simulink model "PI_VSRPhysicalModel"  (R2021a)
settings: Solver=ode23  StartTime=0.0  StopTime=.2  FixedStep=1e-6  MaxStep=1e-6  RelTol=1e-3
InitFcn:
  | Ts = 1e-6;
  | f_PWM = 20000;
  | tf = f_PWM * Ts;
  | L = 2e-3;
  | omega = 2*pi*50;
  | a = exp(1i*2*pi/3);
  | R = 0.5;
  | C  = 1500e-6;
  | tau_c = 7.95e-05;
  | kp = L/tau_c;
  | ki = R/tau_c;
undefined symbols (not defined in the file): DiscIntNeverNeededParam
libraries: pid_lib x5, spsabctodq0Lib x4, spsControlledVoltageSourceLib x3, spsSeriesRLCBranchLib x2, spsdq0toAlphaBetaZeroLib x2, spsGroundLib x1, spsThreePhaseVIMeasurementLib x1, simulink x1, mcbcontrolslib x1, spsThreePhaseSeriesRLCBranchLib x1, spsUniversalBridgeLib x1, spsVoltageMeasurementLib x1
settings Model: Creator=Kibrom  LastModifiedBy=Kibrom

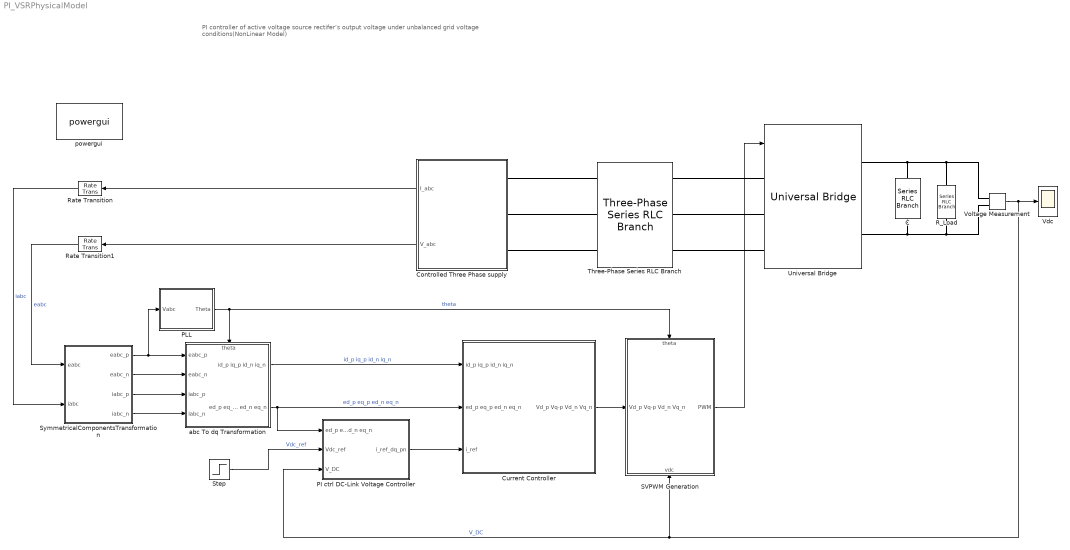
== system PI_VSRPhysicalModel ==
  note: PI controller of active voltage source rectifer’s output voltage under unbalanced grid voltage conditions(NonLinear Model)
  C : spsSeriesRLCBranchLib/Series RLC Branch  LConnTagsString=__new0  RConnTagsString=__new0  BranchType=C  Resistance=1  Inductance=1e-3  SetiL0=off  InitialCurrent=0  Capacitance=1500e-6  Setx0=on  InitialVoltage=650  Measurements=None
  Controlled Three Phase supply : Subsystem
      settings: PortSchema="{\"entries\":[{\"content\":{\"sides\":[{\"content\":{\"connectorIds\":[\"Out1\",\"Out2\"]},\"type\":\"ConnectorPlacement.EquallySpacedRectSide\",\"uuid\":\"e5d84f7a-0d8d-41f6-8cc2-6d81f08370fc\"},{\"content\":{\"connectorIds\":[\"RConn1\",\"RConn2\",\"RConn3\"],\"side\":\"RIGHT\"},\"type\":\"ConnectorPlacement.EquallySpacedRectSide\",\"uuid\":\"372d453a-1c29-4369-a80d-bd12301de137\"},{\"content\":{\"connectorIds\":[],\"side\":\"TOP\"},\"type\":\"ConnectorPlacement.EquallySpacedRectSide\",\"uuid\":\"f7f34885-8130-4d5d-8b71-b12e9f31364c\"}]},\"type\":\"ConnectorPlacement.EquallySpacedConnector\",\"uuid\":\"3797b9c2-a6ae-4ab8-888b-5dd066a2b1e3\"}],\"packageUris\":[\"http://schema.mathworks.com/mf0/Connector/R2020b\"],\"version\":\"1.0\"}"
  Current Controller : Subsystem
  PI ctrl DC-Link Voltage Controller : Subsystem
  PLL : Subsystem
  R_Load : spsSeriesRLCBranchLib/Series RLC Branch  LConnTagsString=__new0  RConnTagsString=__new0  BranchType=R  Resistance=60  Inductance=1e-3  SetiL0=off  InitialCurrent=0  Capacitance=1e-6  Setx0=off  InitialVoltage=0  Measurements=None
  Rate Transition : RateTransition  OutPortSampleTime=5e-5
  Rate Transition1 : RateTransition  OutPortSampleTime=5e-5
  SVPWM Generation : Subsystem
      settings: PortSchema="{\"entries\":[{\"content\":{\"sides\":[{\"content\":{\"connectorIds\":[\"In1\"]},\"type\":\"ConnectorPlacement.EquallySpacedRectSide\",\"uuid\":\"b01bcb52-9446-408f-a811-167d66cc3532\"},{\"content\":{\"connectorIds\":[\"Out1\"],\"side\":\"RIGHT\"},\"type\":\"ConnectorPlacement.EquallySpacedRectSide\",\"uuid\":\"648c50fb-9991-4e3a-92fd-e8050aaa738b\"},{\"content\":{\"connectorIds\":[\"In2\"],\"side\":\"TOP\"},\"type\":\"ConnectorPlacement.EquallySpacedRectSide\",\"uuid\":\"7ec30d75-e250-4e03-a8de-fbe51cb0d640\"},{\"content\":{\"connectorIds\":[\"In3\"],\"side\":\"BOTTOM\"},\"type\":\"ConnectorPlacement.EquallySpacedRectSide\",\"uuid\":\"2bac38e0-cfd2-4a7e-a696-b4a008d5ca86\"}]},\"type\":\"ConnectorPlacement.EquallySpacedConnector\",\"uuid\":\"00db0e70-35b6-41ae-bea5-41b2b525dd01\"}],\"packageUris\":[\"http://schema.mathworks.com/mf0/Connector/R2020b\"],\"version\":\"1.0\"}"
  Step : Step  Time=0.1  Before=650  After=700  SampleTime=5e-04
  SymmetricalComponentsTransformation : Subsystem
  Three-Phase Series RLC Branch : spsThreePhaseSeriesRLCBranchLib/Three-Phase Series RLC Branch  LConnTagsString=A|B|C  RConnTagsString=A|B|C  BranchType=RL  Resistance=R  Inductance=2*L  Capacitance=1e-6  Measurements=None
  Universal Bridge : spsUniversalBridgeLib/Universal Bridge  Arms=3  SnubberResistance=1e5  SnubberCapacitance=inf  Device=IGBT / Diodes  Ron=1e-3  Lon=0  ForwardVoltages="[  0  0  ]"  ForwardVoltage=0  GTOparameters=[ 10e-6 , 20e-6 ]  IGBTparameters=[ 1e-6 , 2e-6 ]  Measurements=None  Measurements_2=None  converterType=Rectifier
  Vdc : Scope
  Voltage Measurement : spsVoltageMeasurementLib/Voltage Measurement  PhasorSimulation=off  OutputType=Complex  PSBequivalent=0
  abc To dq Transformation : Subsystem
      settings: PortSchema="{\"entries\":[{\"content\":{\"sides\":[{\"content\":{\"connectorIds\":[\"In1\",\"In2\",\"In3\",\"In4\"]},\"type\":\"ConnectorPlacement.EquallySpacedRectSide\",\"uuid\":\"dcaee8e7-dac1-4a7e-bdf9-5644c9a478e5\"},{\"content\":{\"connectorIds\":[\"Out1\",\"Out2\"],\"side\":\"RIGHT\"},\"type\":\"ConnectorPlacement.EquallySpacedRectSide\",\"uuid\":\"35135458-27d9-4a99-822f-710c0f77fa66\"},{\"content\":{\"connectorIds\":[\"In5\"],\"side\":\"TOP\"},\"type\":\"ConnectorPlacement.EquallySpacedRectSide\",\"uuid\":\"74ffbf0c-7c15-41c6-8afa-503588a6e7a3\"}]},\"type\":\"ConnectorPlacement.EquallySpacedConnector\",\"uuid\":\"51b18d8e-0b4d-44db-b422-35434fbd35e0\"}],\"packageUris\":[\"http://schema.mathworks.com/mf0/Connector/R2020b\"],\"version\":\"1.0\"}"
  powergui : spspowerguiLib/powergui  Priority=1  SimulationMode=Discrete  SampleTime=Ts  frequency=60  Iterations=50  frequencyindice=0  Pbase=100e6  ErrMax=1e-4  UnitsV=kV  UnitsW=MW  buscounter=0  FunctionMessages=off  echomessages=off  EnableUseOfTLC=off  CurrentSourceSwitches=off  DisableSnubberDevices=off  DisableRonSwitches=off  DisableVfSwitches=off  DisplayEquations=off  AutomaticDiscreteSolvers=off  SolverType=Tustin/Backward Euler (TBE)  Interpol=off  ExternalGateDelay=off  methode=off  Ts=100  x0status=blocks  SPID=on  SwTol=0  HookPort=off  NonlinearTolerance=1e-4  nMaxIteration=100  ContinueOnMaxIteration=off  RestoreLinks=warning  ResistiveCurrentMeasurement=off  Frange=[0:2:500]  Ylog=off  Xlog=on  ShowGrid=off  save=off  variable=ZData  structure=0  ZoomFFT=off  StartTime=0.0  cycles=1  DisplayStyle=1  fundamental=60  FreqAxis=off  MaxFrequency=1000  frequencyindicesteady=1  RmsSteady=1  display=off
  wires:
  SVPWM Generation/1(PWM) -> Universal Bridge/1
  PLL/1(Theta) -> SVPWM Generation/2(theta), abc To dq Transformation/5(theta)  "theta"
  Voltage Measurement/1 -> PI ctrl DC-Link Voltage Controller/3(V_DC), SVPWM Generation/3(vdc), Vdc/1  "V_DC"
  Rate Transition1/1 -> SymmetricalComponentsTransformation/1(eabc)  "eabc"
  Current Controller/1(Vd_p Vq-p Vd_n Vq_n) -> SVPWM Generation/1(Vd_p Vq-p Vd_n Vq_n)
  abc To dq Transformation/1(id_p iq_p id_n iq_n) -> Current Controller/1(id_p iq_p id_n iq_n)  "id_p iq_p id_n iq_n"
  abc To dq Transformation/2(ed_p eq_p ed_n eq_n) -> PI ctrl DC-Link Voltage Controller/1(ed_p eq_p ed_n eq_n), Current Controller/2(ed_p eq_p ed_n eq_n)  "ed_p eq_p ed_n eq_n"
  Rate Transition/1 -> SymmetricalComponentsTransformation/2(iabc)  "iabc"
  Controlled Three Phase supply/1(I_abc) -> Rate Transition/1
  Controlled Three Phase supply/2(V_abc) -> Rate Transition1/1
  SymmetricalComponentsTransformation/1(eabc_p) -> PLL/1(Vabc), abc To dq Transformation/1(eabc_p)
  SymmetricalComponentsTransformation/4(iabc_n) -> abc To dq Transformation/4(iabc_n)
  SymmetricalComponentsTransformation/3(iabc_p) -> abc To dq Transformation/3(iabc_p)
  SymmetricalComponentsTransformation/2(eabc_n) -> abc To dq Transformation/2(eabc_n)
  Step/1 -> PI ctrl DC-Link Voltage Controller/2(Vdc_ref)  "Vdc_ref"
  PI ctrl DC-Link Voltage Controller/1(i_ref_dq_pn) -> Current Controller/3(i_ref)
  connections:
  Voltage Measurement/LConn2 -- Universal Bridge/RConn2 -- C/RConn1 -- R_Load/RConn1
  Universal Bridge/LConn1 -- Three-Phase Series RLC Branch/RConn1
  Universal Bridge/LConn2 -- Three-Phase Series RLC Branch/RConn2
  Universal Bridge/LConn3 -- Three-Phase Series RLC Branch/RConn3
  Universal Bridge/RConn1 -- R_Load/LConn1 -- Voltage Measurement/LConn1 -- C/LConn1
  Controlled Three Phase supply/RConn1 -- Three-Phase Series RLC Branch/LConn1
  Controlled Three Phase supply/RConn2 -- Three-Phase Series RLC Branch/LConn2
  Controlled Three Phase supply/RConn3 -- Three-Phase Series RLC Branch/LConn3

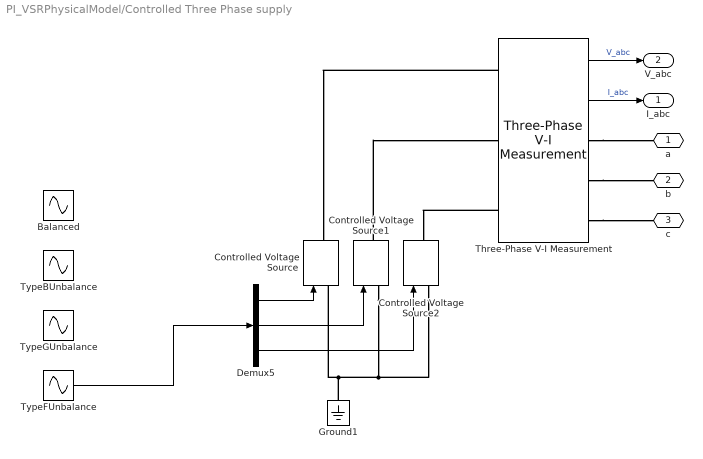
== system PI_VSRPhysicalModel/Controlled Three Phase supply ==
  Balanced : Sin  Amplitude=sqrt(2)*[230 230 230]  Frequency=2*pi*50  Phase=[0 240 120]*(pi/180)  SampleTime=0
  Controlled Voltage Source : spsControlledVoltageSourceLib/Controlled Voltage Source  Initialize=on  Source_Type=AC  Amplitude=0  Phase=0  Frequency=0  Measurements=None
  Controlled Voltage Source1 : spsControlledVoltageSourceLib/Controlled Voltage Source  Initialize=on  Source_Type=AC  Amplitude=0  Phase=0  Frequency=0  Measurements=None
  Controlled Voltage Source2 : spsControlledVoltageSourceLib/Controlled Voltage Source  Initialize=on  Source_Type=AC  Amplitude=0  Phase=0  Frequency=0  Measurements=None
  Demux5 : Demux  Outputs=3
  Ground1 : spsGroundLib/Ground  LConnTagsString=a
  Three-Phase V-I Measurement : spsThreePhaseVIMeasurementLib/Three-Phase V-I Measurement  VoltageMeasurement=phase-to-ground  SetLabelV=off  LabelV=Vabc  Vpu=off  VpuLL=off  CurrentMeasurement=yes  SetLabelI=off  LabelI=Iabc  Ipu=off  Pbase=100e6  Vbase=500e3  OutputType=Complex  PhasorSimulation=off  PSBequivalent=0
  TypeBUnbalance : Sin  Amplitude=sqrt(2)*[185 230 230]  Frequency=2*pi*50  Phase=[0 240 120]*(pi/180)  SampleTime=0
  TypeFUnbalance : Sin  Amplitude=sqrt(2)*[184 207.4 207.4]  Frequency=2*pi*50  Phase=[0 243.7 116.3]*(pi/180)  SampleTime=0
  TypeGUnbalance : Sin  Amplitude=sqrt(2)*[214.6 192.1 192.1]  Frequency=2*pi*50  Phase=[0 236 124]*(pi/180)  SampleTime=0
  a : PMIOPort  Side=Right
  b : PMIOPort  Port=2  Side=Right
  c : PMIOPort  Port=3  Side=Right
  I_abc : Outport
  V_abc : Outport  Port=2
  wires:
  TypeFUnbalance/1 -> Demux5/1
  Three-Phase V-I Measurement/2 -> I_abc/1  "I_abc"
  Demux5/2 -> Controlled Voltage Source1/1
  Demux5/3 -> Controlled Voltage Source2/1
  Demux5/1 -> Controlled Voltage Source/1
  Three-Phase V-I Measurement/1 -> V_abc/1  "V_abc"
  connections:
  Controlled Voltage Source1/RConn1 -- Three-Phase V-I Measurement/LConn2
  Controlled Voltage Source/LConn1 -- Ground1/LConn1 -- Controlled Voltage Source1/LConn1 -- Controlled Voltage Source2/LConn1
  Three-Phase V-I Measurement/LConn3 -- Controlled Voltage Source2/RConn1
  Three-Phase V-I Measurement/LConn1 -- Controlled Voltage Source/RConn1
  Three-Phase V-I Measurement/RConn3 -- c/RConn1
  Three-Phase V-I Measurement/RConn1 -- a/RConn1
  Three-Phase V-I Measurement/RConn2 -- b/RConn1

== system PI_VSRPhysicalModel/Current Controller ==
  id_p iq_p id_n iq_n : Inport
  ed_p eq_p ed_n eq_n : Inport  Port=2
  i_ref : Inport  Port=3
  Demux : Demux
  Demux1 : Demux  Outputs=2
  Demux2 : Demux  Outputs=2
  Mux : Mux
  NegatveSeq Current Controller : Subsystem
      settings: PortSchema="{\"entries\":[{\"content\":{\"sides\":[{\"content\":{\"connectorIds\":[\"In1\",\"In2\",\"In3\"]},\"type\":\"ConnectorPlacement.EquallySpacedRectSide\",\"uuid\":\"2bdf4aa8-c3f9-436b-9835-043d932fea71\"},{\"content\":{\"connectorIds\":[\"Out1\",\"Out2\"],\"side\":\"RIGHT\"},\"type\":\"ConnectorPlacement.EquallySpacedRectSide\",\"uuid\":\"c965a7a2-5936-47cc-8492-850bd324378e\"},{\"content\":{\"connectorIds\":[],\"side\":\"TOP\"},\"type\":\"ConnectorPlacement.EquallySpacedRectSide\",\"uuid\":\"45debca4-d3b7-48eb-be8d-4eccd646cb24\"},{\"content\":{\"connectorIds\":[\"In4\"],\"side\":\"BOTTOM\"},\"type\":\"ConnectorPlacement.EquallySpacedRectSide\",\"uuid\":\"6975aea9-83b3-4c6b-a4f1-94e60a0e1fe9\"}]},\"type\":\"ConnectorPlacement.EquallySpacedConnector\",\"uuid\":\"b897b5d1-f6c9-41b8-aee6-e6cc6417929b\"}],\"packageUris\":[\"http://schema.mathworks.com/mf0/Connector/R2020b\"],\"version\":\"1.0\"}"
  PostiveSeq Current Controller : Subsystem
      settings: PortSchema="{\"entries\":[{\"content\":{\"sides\":[{\"content\":{\"connectorIds\":[\"In1\",\"In2\",\"In3\"]},\"type\":\"ConnectorPlacement.EquallySpacedRectSide\",\"uuid\":\"2bdf4aa8-c3f9-436b-9835-043d932fea71\"},{\"content\":{\"connectorIds\":[\"Out1\",\"Out2\"],\"side\":\"RIGHT\"},\"type\":\"ConnectorPlacement.EquallySpacedRectSide\",\"uuid\":\"c965a7a2-5936-47cc-8492-850bd324378e\"},{\"content\":{\"connectorIds\":[\"In4\"],\"side\":\"TOP\"},\"type\":\"ConnectorPlacement.EquallySpacedRectSide\",\"uuid\":\"45debca4-d3b7-48eb-be8d-4eccd646cb24\"}]},\"type\":\"ConnectorPlacement.EquallySpacedConnector\",\"uuid\":\"b897b5d1-f6c9-41b8-aee6-e6cc6417929b\"}],\"packageUris\":[\"http://schema.mathworks.com/mf0/Connector/R2020b\"],\"version\":\"1.0\"}"
  Vd_p Vq-p Vd_n Vq_n : Outport
  wires:
  Demux1/1 -> PostiveSeq Current Controller/1(id_p iq_p)  "id_p iq_p"
  Demux/3 -> NegatveSeq Current Controller/1(id_ref)
  Demux2/2 -> NegatveSeq Current Controller/4(ed_n eq_n)  "ed_n eq_n"
  PostiveSeq Current Controller/1(Vd_p) -> Mux/1
  Demux2/1 -> PostiveSeq Current Controller/4(ed_p eq_p)  "ed_p eq_p"
  Demux/4 -> NegatveSeq Current Controller/2(iq_ref)
  NegatveSeq Current Controller/1(Vd_n) -> Mux/3
  NegatveSeq Current Controller/2(Vq_n) -> Mux/4
  Demux/1 -> PostiveSeq Current Controller/2(id_ref)
  Demux/2 -> PostiveSeq Current Controller/3(iq_ref)
  PostiveSeq Current Controller/2(Vq_p) -> Mux/2
  Demux1/2 -> NegatveSeq Current Controller/3(id_n iq_n)  "id_n iq_n"
  Mux/1 -> Vd_p Vq-p Vd_n Vq_n/1  "Vd_p Vq-p Vd_n Vq_n"
  i_ref/1 -> Demux/1
  id_p iq_p id_n iq_n/1 -> Demux1/1
  ed_p eq_p ed_n eq_n/1 -> Demux2/1

== system PI_VSRPhysicalModel/PI ctrl DC-Link Voltage Controller ==
  ed_p eq_p ed_n eq_n : Inport
  Vdc_ref : Inport  Port=2
  V_DC : Inport  Port=3
  MATLAB Function : MATLAB Function  TreatAsAtomicUnit=on
  PID Controller : pid_lib/PID Controller  Controller=PID  Form=Parallel  TimeDomain=Continuous-time  UseExternalTs=off  SampleTime=-1  IntegratorMethod=Forward Euler  FilterMethod=Forward Euler  ControllerParametersSource=internal  P=1  I=1  D=0  UseFilter=on  N=100  TunerSelectOption=Transfer Function Based (PID Tuner App)  InitialConditionSource=internal  InitialConditionForIntegrator=0  InitialConditionForFilter=0  DifferentiatorICPrevScaledInput=0  ExternalReset=none  TrackingMode=off  Kt=1  LimitOutput=off  SatLimitsSource=internal  UpperSaturationLimit=inf  LowerSaturationLimit=-inf  LinearizeAsGain=on  AntiWindupMode=none  Kb=1  POutMin=[]  POutMax=[]  IOutMin=[]  IOutMax=[]  DOutMin=[]  DOutMax=[]  NOutMin=[]  NOutMax=[]  SumOutMin=[]  SumOutMax=[]  SaturationOutMin=[]  SaturationOutMax=[]  PParamMin=[]  PParamMax=[]  IParamMin=[]  IParamMax=[]  DParamMin=[]  DParamMax=[]  NParamMin=[]  NParamMax=[]  KbParamMin=[]  KbParamMax=[]  KtParamMin=[]  KtParamMax=[]  KbOutMin=[]  KbOutMax=[]  KtOutMin=[]  KtOutMax=[]  IntegratorOutMin=[]  IntegratorOutMax=[]  FilterOutMin=[]  FilterOutMax=[]  SumI1OutMin=[]  SumI1OutMax=[]  SumI2OutMin=[]  SumI2OutMax=[]  SumI3OutMin=[]  SumI3OutMax=[]  SumI4OutMin=[]  SumI4OutMax=[]  SumDOutMin=[]  SumDOutMax=[]  DifferentiatorOutMin=[]  DifferentiatorOutMax=[]  FilterDiffOutCoefMin=[]  FilterDiffOutCoefMax=[]  ReciprocalOutMin=[]  ReciprocalOutMax=[]  SumDenOutMin=[]  SumDenOutMax=[]  SumNumOutMin=[]  SumNumOutMax=[]  DivideOutMin=[]  DivideOutMax=[]  UdiffTsProdOutMin=[]  UdiffTsProdOutMax=[]  NTsProdOutMin=[]  NTsProdOutMax=[]  UintegralTsProdOutMin=[]  UintegralTsProdOutMax=[]  UngainTsProdOutMin=[]  UngainTsProdOutMax=[]  IntegratorContinuousStateAttributes=''  IntegratorStateMustResolveToSignalObject=off  IntegratorRTWStateStorageClass=Auto  FilterContinuousStateAttributes=''  FilterStateMustResolveToSignalObject=off  FilterRTWStateStorageClass=Auto  ParallelPVariant=InternalParameters  IdealPVariant=Disabled  IVariant=InternalParameters  DVariant=InternalParameters  IntegratorVariant=Continuous  SatVariant=Disabled  AWVariant=Passthrough  PCopyVariant=Disabled  TRVariant=Disabled  FdbkBlocksVariant=Forward  IdealPFdbkVariant=Disabled  SatFdbkVariant=Disabled  DerivativeFilterVariant=ContFilter  NVariant=InternalParameters  NCopyVariant=Disabled  FilterICVariant=InternalICsFilter  IntegratorICVariant=InternalICs  ExternalResetVariant=Disabled  TRSumVariant=Passthrough  SumFdbkVariant=Disabled  SumVariant=Sum_PID  TsampFilterVariant=InternalTs  TsampNgainVariant=Passthrough  TsampIntegralVariant=Passthrough  ExternalSaturationOutDataTypeStr=Inherit: Same as second input
  Product : Product
  Rate Transition2 : RateTransition  OutPortSampleTime=5e-04
  Rate Transition3 : RateTransition  OutPortSampleTime=5e-04
  Sum : Sum  Inputs=|++
  i_ref_dq_pn : Outport
  wires:
  Rate Transition3/1 -> Sum/2
  ed_p eq_p ed_n eq_n/1 -> Rate Transition2/1
  Product/1 -> MATLAB Function/2(wref)
  Sum/1 -> PID Controller/1
  PID Controller/1 -> Product/2
  Vdc_ref/1 -> Product/1, Sum/1
  Rate Transition2/1 -> MATLAB Function/1(Grid_Voltages)
  V_DC/1 -> Rate Transition3/1
  MATLAB Function/1(i_ref) -> i_ref_dq_pn/1  "i_ref_dq_pn"

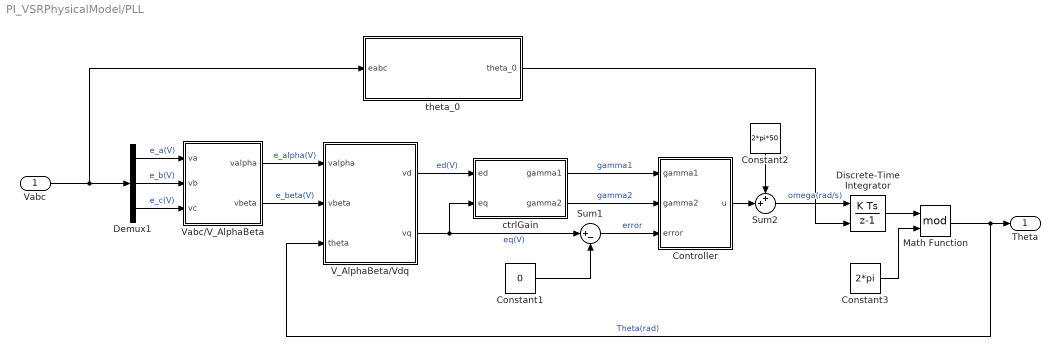
== system PI_VSRPhysicalModel/PLL ==
  Vabc : Inport
  Constant1 : Constant  Value=0
  Constant2 : Constant  Value=2*pi*50
  Constant3 : Constant  Value=2*pi
  Controller : Subsystem
  Demux1 : Demux  Outputs=3
  Discrete-Time Integrator : DiscreteIntegrator  InitialConditionSource=external  SampleTime=5e-5  ICPrevOutput=DiscIntNeverNeededParam  ICPrevScaledInput=DiscIntNeverNeededParam
  Math Function : Math  Operator=mod  SaturateOnIntegerOverflow=on
  Sum1 : Sum  Inputs=|+-
  Sum2 : Sum  Inputs=++|
  V_AlphaBeta/Vdq : MATLAB Function  TreatAsAtomicUnit=on
  Vabc/V_AlphaBeta : MATLAB Function  TreatAsAtomicUnit=on
  ctrlGain : MATLAB Function  TreatAsAtomicUnit=on
  theta_0 : Subsystem
  Theta : Outport
  wires:
  Demux1/2 -> Vabc/V_AlphaBeta/2(vb)  "e_b(V)"
  Demux1/3 -> Vabc/V_AlphaBeta/3(vc)  "e_c(V)"
  Demux1/1 -> Vabc/V_AlphaBeta/1(va)  "e_a(V)"
  Vabc/V_AlphaBeta/2(vbeta) -> V_AlphaBeta/Vdq/2(vbeta)  "e_beta(V)"
  Vabc/V_AlphaBeta/1(valpha) -> V_AlphaBeta/Vdq/1(valpha)  "e_alpha(V)"
  V_AlphaBeta/Vdq/2(vq) -> ctrlGain/2(eq), Sum1/1  "eq(V)"
  Constant1/1 -> Sum1/2
  Constant2/1 -> Sum2/1
  Sum2/1 -> Discrete-Time Integrator/1  "omega(rad/s)"
  Discrete-Time Integrator/1 -> Math Function/1
  V_AlphaBeta/Vdq/1(vd) -> ctrlGain/1(ed)  "ed(V)"
  ctrlGain/1(gamma1) -> Controller/1(gamma1)  "gamma1"
  ctrlGain/2(gamma2) -> Controller/2(gamma2)  "gamma2"
  Sum1/1 -> Controller/3(error)  "error"
  Controller/1(u) -> Sum2/2
  Math Function/1 -> Theta/1, V_AlphaBeta/Vdq/3(theta)  "Theta(rad)"
  Constant3/1 -> Math Function/2
  Vabc/1 -> theta_0/1(eabc), Demux1/1
  theta_0/1(theta_0) -> Discrete-Time Integrator/2

== system PI_VSRPhysicalModel/SVPWM Generation ==
  Vd_p Vq-p Vd_n Vq_n : Inport
  theta : Inport  Port=2
  vdc : Inport  Port=3
  Inverse Park Transformation : Subsystem
  PWM Generator : Subsystem
  Saturation Block : Subsystem
  Space Vector Generator : mcbcontrolslib/Space Vector Generator
      settings: SourceProductBaseCode=MT
  PWM : Outport
  wires:
  theta/1 -> Inverse Park Transformation/1(theta)
  Vd_p Vq-p Vd_n Vq_n/1 -> Inverse Park Transformation/2(Vd_p Vq-p Vd_n Vq_n)  "Vd_p Vq-p Vd_n Vq_n"
  vdc/1 -> Saturation Block/1(vdc)
  Inverse Park Transformation/1(v_alpha v_beta) -> Saturation Block/2(v_alpha v_beta)  "v_alpha v_beta"
  Saturation Block/1(v_alpha) -> Space Vector Generator/1
  Saturation Block/2(v_beta) -> Space Vector Generator/2
  Space Vector Generator/1 -> PWM Generator/1(va0)  "va0"
  Space Vector Generator/2 -> PWM Generator/2(vb0)  "vb0"
  Space Vector Generator/3 -> PWM Generator/3(vc0)  "vc0"
  PWM Generator/1(PWM) -> PWM/1

== system PI_VSRPhysicalModel/SymmetricalComponentsTransformation ==
  eabc : Inport
  iabc : Inport  Port=2
  Current SymmetricalComponentsTransformation : Subsystem
  Terminator : Terminator
  Terminator1 : Terminator
  Voltage SymmetricalComponentsTransformation : Subsystem
  eabc_p : Outport
  eabc_n : Outport  Port=2
  iabc_p : Outport  Port=3
  iabc_n : Outport  Port=4
  wires:
  Current SymmetricalComponentsTransformation/3(Zero) -> Terminator1/1
  Voltage SymmetricalComponentsTransformation/1(Postive) -> eabc_p/1  "eabc_p"
  Voltage SymmetricalComponentsTransformation/3(Zero) -> Terminator/1
  eabc/1 -> Voltage SymmetricalComponentsTransformation/1(X_abc)
  Current SymmetricalComponentsTransformation/1(Postive) -> iabc_p/1  "iabc_p"
  Current SymmetricalComponentsTransformation/2(Negative) -> iabc_n/1  "iabc_n"
  iabc/1 -> Current SymmetricalComponentsTransformation/1(X_abc)
  Voltage SymmetricalComponentsTransformation/2(Negative) -> eabc_n/1  "eabc_n"

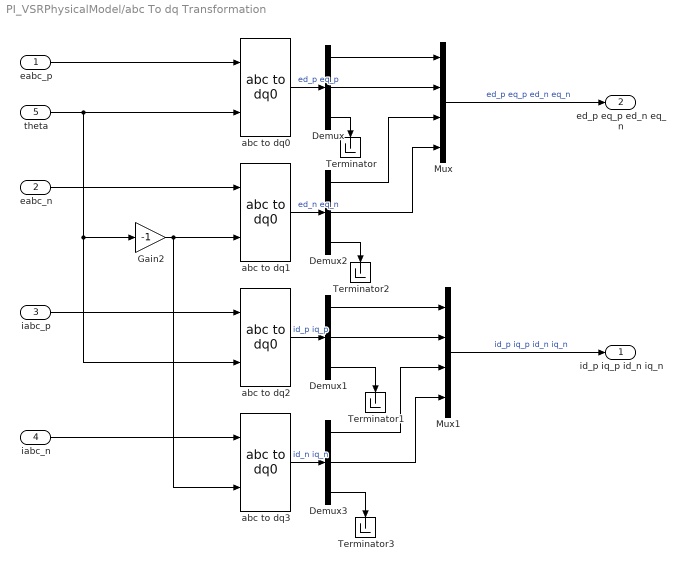
== system PI_VSRPhysicalModel/abc To dq Transformation ==
  eabc_p : Inport
  eabc_n : Inport  Port=2
  iabc_p : Inport  Port=3
  iabc_n : Inport  Port=4
  theta : Inport  Port=5
  Demux{,1..3} (4 alike) : Demux  Outputs=3
  Gain2 : Gain  Gain=-1
  Mux : Mux
  Mux1 : Mux
  Terminator{,1..3} (4 alike) : Terminator
  abc to dq{0..3} (4 alike) : spsabctodq0Lib/abc to dq0  Alignment=Aligned with phase A axis
  id_p iq_p id_n iq_n : Outport
  ed_p eq_p ed_n eq_n : Outport  Port=2
  wires:
  Mux1/1 -> id_p iq_p id_n iq_n/1  "id_p iq_p id_n iq_n"
  iabc_n/1 -> abc to dq3/1
  Gain2/1 -> abc to dq3/2, abc to dq1/2
  theta/1 -> abc to dq2/2, Gain2/1, abc to dq0/2
  iabc_p/1 -> abc to dq2/1
  Mux/1 -> ed_p eq_p ed_n eq_n/1  "ed_p eq_p ed_n eq_n"
  eabc_n/1 -> abc to dq1/1
  eabc_p/1 -> abc to dq0/1
  Demux/1 -> Mux/1
  Demux/2 -> Mux/2
  Demux/3 -> Terminator/1
  abc to dq0/1 -> Demux/1  "ed_p eq_p"
  Demux1/3 -> Terminator1/1
  Demux1/1 -> Mux1/1
  Demux1/2 -> Mux1/2
  abc to dq2/1 -> Demux1/1  "id_p iq_p"
  Demux2/3 -> Terminator2/1
  Demux2/1 -> Mux/3
  Demux2/2 -> Mux/4
  abc to dq1/1 -> Demux2/1  "ed_n eq_n"
  Demux3/3 -> Terminator3/1
  Demux3/1 -> Mux1/3
  Demux3/2 -> Mux1/4
  abc to dq3/1 -> Demux3/1  "id_n iq_n"

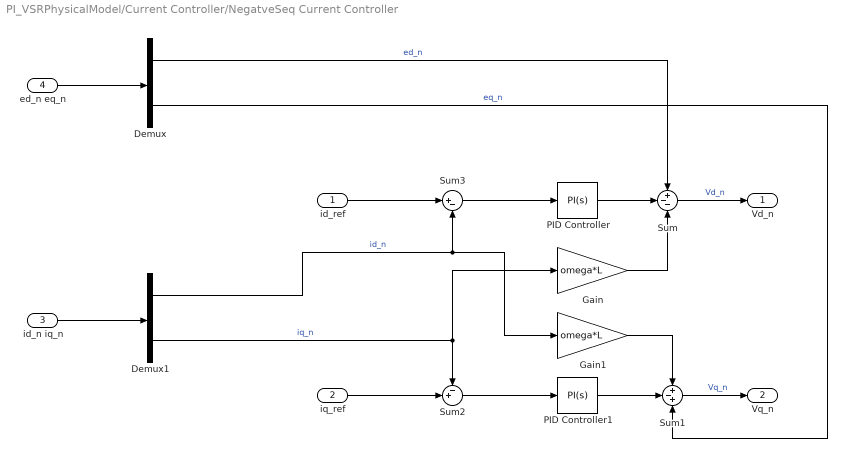
== system PI_VSRPhysicalModel/Current Controller/NegatveSeq Current Controller ==
  id_ref : Inport
  iq_ref : Inport  Port=2
  id_n iq_n : Inport  Port=3
  ed_n eq_n : Inport  Port=4
  Demux : Demux  Outputs=2
  Demux1 : Demux  Outputs=2
  Gain : Gain  Gain=omega*L
  Gain1 : Gain  Gain=omega*L
  PID Controller : pid_lib/PID Controller  Controller=PI  Form=Parallel  TimeDomain=Continuous-time  UseExternalTs=off  SampleTime=-1  IntegratorMethod=Forward Euler  FilterMethod=Forward Euler  ControllerParametersSource=internal  P=kp  I=ki  D=0  UseFilter=on  N=100  TunerSelectOption=Transfer Function Based (PID Tuner App)  InitialConditionSource=internal  InitialConditionForIntegrator=0  InitialConditionForFilter=0  DifferentiatorICPrevScaledInput=0  ExternalReset=none  TrackingMode=off  Kt=1  LimitOutput=off  SatLimitsSource=internal  UpperSaturationLimit=inf  LowerSaturationLimit=-inf  LinearizeAsGain=on  AntiWindupMode=none  Kb=1  POutMin=[]  POutMax=[]  IOutMin=[]  IOutMax=[]  DOutMin=[]  DOutMax=[]  NOutMin=[]  NOutMax=[]  SumOutMin=[]  SumOutMax=[]  SaturationOutMin=[]  SaturationOutMax=[]  PParamMin=[]  PParamMax=[]  IParamMin=[]  IParamMax=[]  DParamMin=[]  DParamMax=[]  NParamMin=[]  NParamMax=[]  KbParamMin=[]  KbParamMax=[]  KtParamMin=[]  KtParamMax=[]  KbOutMin=[]  KbOutMax=[]  KtOutMin=[]  KtOutMax=[]  IntegratorOutMin=[]  IntegratorOutMax=[]  FilterOutMin=[]  FilterOutMax=[]  SumI1OutMin=[]  SumI1OutMax=[]  SumI2OutMin=[]  SumI2OutMax=[]  SumI3OutMin=[]  SumI3OutMax=[]  SumI4OutMin=[]  SumI4OutMax=[]  SumDOutMin=[]  SumDOutMax=[]  DifferentiatorOutMin=[]  DifferentiatorOutMax=[]  FilterDiffOutCoefMin=[]  FilterDiffOutCoefMax=[]  ReciprocalOutMin=[]  ReciprocalOutMax=[]  SumDenOutMin=[]  SumDenOutMax=[]  SumNumOutMin=[]  SumNumOutMax=[]  DivideOutMin=[]  DivideOutMax=[]  UdiffTsProdOutMin=[]  UdiffTsProdOutMax=[]  NTsProdOutMin=[]  NTsProdOutMax=[]  UintegralTsProdOutMin=[]  UintegralTsProdOutMax=[]  UngainTsProdOutMin=[]  UngainTsProdOutMax=[]  IntegratorContinuousStateAttributes=''  IntegratorStateMustResolveToSignalObject=off  IntegratorRTWStateStorageClass=Auto  FilterContinuousStateAttributes=''  FilterStateMustResolveToSignalObject=off  FilterRTWStateStorageClass=Auto  ParallelPVariant=InternalParameters  IdealPVariant=Disabled  IVariant=InternalParameters  DVariant=Disabled  IntegratorVariant=Continuous  SatVariant=Disabled  AWVariant=Passthrough  PCopyVariant=Disabled  TRVariant=Disabled  FdbkBlocksVariant=Forward  IdealPFdbkVariant=Disabled  SatFdbkVariant=Disabled  DerivativeFilterVariant=Disabled  NVariant=Disabled  NCopyVariant=Disabled_SignalSpec  FilterICVariant=Disabled  IntegratorICVariant=InternalICs  ExternalResetVariant=Disabled  TRSumVariant=Passthrough  SumFdbkVariant=Disabled  SumVariant=Sum_PI  TsampFilterVariant=InternalTs  TsampNgainVariant=Passthrough  TsampIntegralVariant=Passthrough  ExternalSaturationOutDataTypeStr=Inherit: Same as second input
  PID Controller1 : pid_lib/PID Controller  Controller=PI  Form=Parallel  TimeDomain=Continuous-time  UseExternalTs=off  SampleTime=-1  IntegratorMethod=Forward Euler  FilterMethod=Forward Euler  ControllerParametersSource=internal  P=kp  I=ki  D=0  UseFilter=on  N=100  TunerSelectOption=Transfer Function Based (PID Tuner App)  InitialConditionSource=internal  InitialConditionForIntegrator=0  InitialConditionForFilter=0  DifferentiatorICPrevScaledInput=0  ExternalReset=none  TrackingMode=off  Kt=1  LimitOutput=off  SatLimitsSource=internal  UpperSaturationLimit=inf  LowerSaturationLimit=-inf  LinearizeAsGain=on  AntiWindupMode=none  Kb=1  POutMin=[]  POutMax=[]  IOutMin=[]  IOutMax=[]  DOutMin=[]  DOutMax=[]  NOutMin=[]  NOutMax=[]  SumOutMin=[]  SumOutMax=[]  SaturationOutMin=[]  SaturationOutMax=[]  PParamMin=[]  PParamMax=[]  IParamMin=[]  IParamMax=[]  DParamMin=[]  DParamMax=[]  NParamMin=[]  NParamMax=[]  KbParamMin=[]  KbParamMax=[]  KtParamMin=[]  KtParamMax=[]  KbOutMin=[]  KbOutMax=[]  KtOutMin=[]  KtOutMax=[]  IntegratorOutMin=[]  IntegratorOutMax=[]  FilterOutMin=[]  FilterOutMax=[]  SumI1OutMin=[]  SumI1OutMax=[]  SumI2OutMin=[]  SumI2OutMax=[]  SumI3OutMin=[]  SumI3OutMax=[]  SumI4OutMin=[]  SumI4OutMax=[]  SumDOutMin=[]  SumDOutMax=[]  DifferentiatorOutMin=[]  DifferentiatorOutMax=[]  FilterDiffOutCoefMin=[]  FilterDiffOutCoefMax=[]  ReciprocalOutMin=[]  ReciprocalOutMax=[]  SumDenOutMin=[]  SumDenOutMax=[]  SumNumOutMin=[]  SumNumOutMax=[]  DivideOutMin=[]  DivideOutMax=[]  UdiffTsProdOutMin=[]  UdiffTsProdOutMax=[]  NTsProdOutMin=[]  NTsProdOutMax=[]  UintegralTsProdOutMin=[]  UintegralTsProdOutMax=[]  UngainTsProdOutMin=[]  UngainTsProdOutMax=[]  IntegratorContinuousStateAttributes=''  IntegratorStateMustResolveToSignalObject=off  IntegratorRTWStateStorageClass=Auto  FilterContinuousStateAttributes=''  FilterStateMustResolveToSignalObject=off  FilterRTWStateStorageClass=Auto  ParallelPVariant=InternalParameters  IdealPVariant=Disabled  IVariant=InternalParameters  DVariant=Disabled  IntegratorVariant=Continuous  SatVariant=Disabled  AWVariant=Passthrough  PCopyVariant=Disabled  TRVariant=Disabled  FdbkBlocksVariant=Forward  IdealPFdbkVariant=Disabled  SatFdbkVariant=Disabled  DerivativeFilterVariant=Disabled  NVariant=Disabled  NCopyVariant=Disabled_SignalSpec  FilterICVariant=Disabled  IntegratorICVariant=InternalICs  ExternalResetVariant=Disabled  TRSumVariant=Passthrough  SumFdbkVariant=Disabled  SumVariant=Sum_PI  TsampFilterVariant=InternalTs  TsampNgainVariant=Passthrough  TsampIntegralVariant=Passthrough  ExternalSaturationOutDataTypeStr=Inherit: Same as second input
  Sum : Sum  Inputs=+--
  Sum1 : Sum  Inputs=+-+
  Sum2 : Sum  Inputs=-+|
  Sum3 : Sum  Inputs=|+-
  Vd_n : Outport
  Vq_n : Outport  Port=2
  wires:
  Sum/1 -> Vd_n/1  "Vd_n"
  Sum1/1 -> Vq_n/1  "Vq_n"
  id_ref/1 -> Sum3/1
  Sum3/1 -> PID Controller/1
  iq_ref/1 -> Sum2/2
  Demux/1 -> Sum/1  "ed_n"
  Gain1/1 -> Sum1/1
  PID Controller/1 -> Sum/2
  PID Controller1/1 -> Sum1/2
  Gain/1 -> Sum/3
  Sum2/1 -> PID Controller1/1
  Demux/2 -> Sum1/3  "eq_n"
  ed_n eq_n/1 -> Demux/1
  id_n iq_n/1 -> Demux1/1
  Demux1/2 -> Gain/1, Sum2/1  "iq_n"
  Demux1/1 -> Gain1/1, Sum3/2  "id_n"

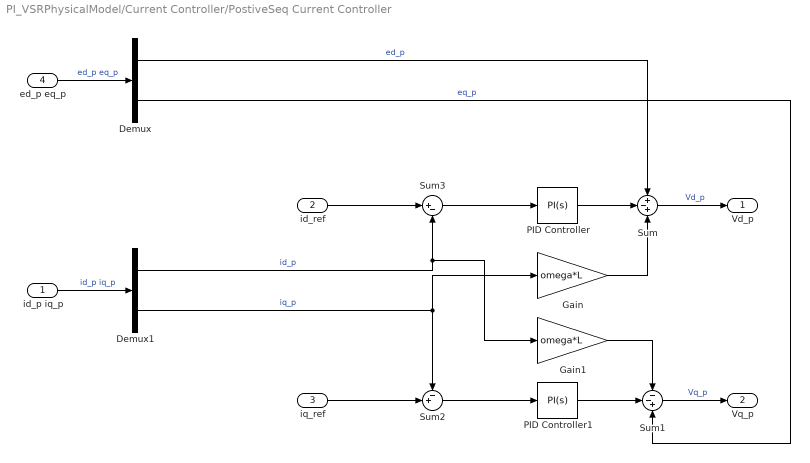
== system PI_VSRPhysicalModel/Current Controller/PostiveSeq Current Controller ==
  id_p iq_p : Inport
  id_ref : Inport  Port=2
  iq_ref : Inport  Port=3
  ed_p eq_p : Inport  Port=4
  Demux : Demux  Outputs=2
  Demux1 : Demux  Outputs=2
  Gain : Gain  Gain=omega*L
  Gain1 : Gain  Gain=omega*L
  PID Controller : pid_lib/PID Controller  Controller=PI  Form=Parallel  TimeDomain=Continuous-time  UseExternalTs=off  SampleTime=-1  IntegratorMethod=Forward Euler  FilterMethod=Forward Euler  ControllerParametersSource=internal  P=kp  I=ki  D=0  UseFilter=on  N=100  TunerSelectOption=Transfer Function Based (PID Tuner App)  InitialConditionSource=internal  InitialConditionForIntegrator=0  InitialConditionForFilter=0  DifferentiatorICPrevScaledInput=0  ExternalReset=none  TrackingMode=off  Kt=1  LimitOutput=off  SatLimitsSource=internal  UpperSaturationLimit=inf  LowerSaturationLimit=-inf  LinearizeAsGain=on  AntiWindupMode=none  Kb=1  POutMin=[]  POutMax=[]  IOutMin=[]  IOutMax=[]  DOutMin=[]  DOutMax=[]  NOutMin=[]  NOutMax=[]  SumOutMin=[]  SumOutMax=[]  SaturationOutMin=[]  SaturationOutMax=[]  PParamMin=[]  PParamMax=[]  IParamMin=[]  IParamMax=[]  DParamMin=[]  DParamMax=[]  NParamMin=[]  NParamMax=[]  KbParamMin=[]  KbParamMax=[]  KtParamMin=[]  KtParamMax=[]  KbOutMin=[]  KbOutMax=[]  KtOutMin=[]  KtOutMax=[]  IntegratorOutMin=[]  IntegratorOutMax=[]  FilterOutMin=[]  FilterOutMax=[]  SumI1OutMin=[]  SumI1OutMax=[]  SumI2OutMin=[]  SumI2OutMax=[]  SumI3OutMin=[]  SumI3OutMax=[]  SumI4OutMin=[]  SumI4OutMax=[]  SumDOutMin=[]  SumDOutMax=[]  DifferentiatorOutMin=[]  DifferentiatorOutMax=[]  FilterDiffOutCoefMin=[]  FilterDiffOutCoefMax=[]  ReciprocalOutMin=[]  ReciprocalOutMax=[]  SumDenOutMin=[]  SumDenOutMax=[]  SumNumOutMin=[]  SumNumOutMax=[]  DivideOutMin=[]  DivideOutMax=[]  UdiffTsProdOutMin=[]  UdiffTsProdOutMax=[]  NTsProdOutMin=[]  NTsProdOutMax=[]  UintegralTsProdOutMin=[]  UintegralTsProdOutMax=[]  UngainTsProdOutMin=[]  UngainTsProdOutMax=[]  IntegratorContinuousStateAttributes=''  IntegratorStateMustResolveToSignalObject=off  IntegratorRTWStateStorageClass=Auto  FilterContinuousStateAttributes=''  FilterStateMustResolveToSignalObject=off  FilterRTWStateStorageClass=Auto  ParallelPVariant=InternalParameters  IdealPVariant=Disabled  IVariant=InternalParameters  DVariant=Disabled  IntegratorVariant=Continuous  SatVariant=Disabled  AWVariant=Passthrough  PCopyVariant=Disabled  TRVariant=Disabled  FdbkBlocksVariant=Forward  IdealPFdbkVariant=Disabled  SatFdbkVariant=Disabled  DerivativeFilterVariant=Disabled  NVariant=Disabled  NCopyVariant=Disabled_SignalSpec  FilterICVariant=Disabled  IntegratorICVariant=InternalICs  ExternalResetVariant=Disabled  TRSumVariant=Passthrough  SumFdbkVariant=Disabled  SumVariant=Sum_PI  TsampFilterVariant=InternalTs  TsampNgainVariant=Passthrough  TsampIntegralVariant=Passthrough  ExternalSaturationOutDataTypeStr=Inherit: Same as second input
  PID Controller1 : pid_lib/PID Controller  Controller=PI  Form=Parallel  TimeDomain=Continuous-time  UseExternalTs=off  SampleTime=-1  IntegratorMethod=Forward Euler  FilterMethod=Forward Euler  ControllerParametersSource=internal  P=kp  I=ki  D=0  UseFilter=on  N=100  TunerSelectOption=Transfer Function Based (PID Tuner App)  InitialConditionSource=internal  InitialConditionForIntegrator=0  InitialConditionForFilter=0  DifferentiatorICPrevScaledInput=0  ExternalReset=none  TrackingMode=off  Kt=1  LimitOutput=off  SatLimitsSource=internal  UpperSaturationLimit=inf  LowerSaturationLimit=-inf  LinearizeAsGain=on  AntiWindupMode=none  Kb=1  POutMin=[]  POutMax=[]  IOutMin=[]  IOutMax=[]  DOutMin=[]  DOutMax=[]  NOutMin=[]  NOutMax=[]  SumOutMin=[]  SumOutMax=[]  SaturationOutMin=[]  SaturationOutMax=[]  PParamMin=[]  PParamMax=[]  IParamMin=[]  IParamMax=[]  DParamMin=[]  DParamMax=[]  NParamMin=[]  NParamMax=[]  KbParamMin=[]  KbParamMax=[]  KtParamMin=[]  KtParamMax=[]  KbOutMin=[]  KbOutMax=[]  KtOutMin=[]  KtOutMax=[]  IntegratorOutMin=[]  IntegratorOutMax=[]  FilterOutMin=[]  FilterOutMax=[]  SumI1OutMin=[]  SumI1OutMax=[]  SumI2OutMin=[]  SumI2OutMax=[]  SumI3OutMin=[]  SumI3OutMax=[]  SumI4OutMin=[]  SumI4OutMax=[]  SumDOutMin=[]  SumDOutMax=[]  DifferentiatorOutMin=[]  DifferentiatorOutMax=[]  FilterDiffOutCoefMin=[]  FilterDiffOutCoefMax=[]  ReciprocalOutMin=[]  ReciprocalOutMax=[]  SumDenOutMin=[]  SumDenOutMax=[]  SumNumOutMin=[]  SumNumOutMax=[]  DivideOutMin=[]  DivideOutMax=[]  UdiffTsProdOutMin=[]  UdiffTsProdOutMax=[]  NTsProdOutMin=[]  NTsProdOutMax=[]  UintegralTsProdOutMin=[]  UintegralTsProdOutMax=[]  UngainTsProdOutMin=[]  UngainTsProdOutMax=[]  IntegratorContinuousStateAttributes=''  IntegratorStateMustResolveToSignalObject=off  IntegratorRTWStateStorageClass=Auto  FilterContinuousStateAttributes=''  FilterStateMustResolveToSignalObject=off  FilterRTWStateStorageClass=Auto  ParallelPVariant=InternalParameters  IdealPVariant=Disabled  IVariant=InternalParameters  DVariant=Disabled  IntegratorVariant=Continuous  SatVariant=Disabled  AWVariant=Passthrough  PCopyVariant=Disabled  TRVariant=Disabled  FdbkBlocksVariant=Forward  IdealPFdbkVariant=Disabled  SatFdbkVariant=Disabled  DerivativeFilterVariant=Disabled  NVariant=Disabled  NCopyVariant=Disabled_SignalSpec  FilterICVariant=Disabled  IntegratorICVariant=InternalICs  ExternalResetVariant=Disabled  TRSumVariant=Passthrough  SumFdbkVariant=Disabled  SumVariant=Sum_PI  TsampFilterVariant=InternalTs  TsampNgainVariant=Passthrough  TsampIntegralVariant=Passthrough  ExternalSaturationOutDataTypeStr=Inherit: Same as second input
  Sum : Sum  Inputs=+-+
  Sum1 : Sum  Inputs=--+
  Sum2 : Sum  Inputs=-+|
  Sum3 : Sum  Inputs=|+-
  Vd_p : Outport
  Vq_p : Outport  Port=2
  wires:
  Demux/2 -> Sum1/3  "eq_p"
  Sum2/1 -> PID Controller1/1
  Gain/1 -> Sum/3
  PID Controller1/1 -> Sum1/2
  PID Controller/1 -> Sum/2
  Gain1/1 -> Sum1/1
  Demux/1 -> Sum/1  "ed_p"
  iq_ref/1 -> Sum2/2
  Sum3/1 -> PID Controller/1
  id_ref/1 -> Sum3/1
  Sum1/1 -> Vq_p/1  "Vq_p"
  Sum/1 -> Vd_p/1  "Vd_p"
  ed_p eq_p/1 -> Demux/1  "ed_p eq_p"
  Demux1/2 -> Gain/1, Sum2/1  "iq_p"
  Demux1/1 -> Sum3/2, Gain1/1  "id_p"
  id_p iq_p/1 -> Demux1/1  "id_p iq_p"

== system PI_VSRPhysicalModel/PLL/Controller ==
  gamma1 : Inport
  gamma2 : Inport  Port=2
  error : Inport  Port=3
  Discrete-Time Integrator : DiscreteIntegrator  SampleTime=5e-5  ICPrevOutput=DiscIntNeverNeededParam  ICPrevScaledInput=DiscIntNeverNeededParam
  Product : Product
  Product1 : Product
  Sum3 : Sum  Inputs=++|
  u : Outport
  wires:
  Product1/1 -> Sum3/2
  Product/1 -> Discrete-Time Integrator/1
  error/1 -> Product1/2, Product/2
  gamma2/1 -> Product1/1  "kp"
  Sum3/1 -> u/1  "u"
  Discrete-Time Integrator/1 -> Sum3/1
  gamma1/1 -> Product/1  "ki"

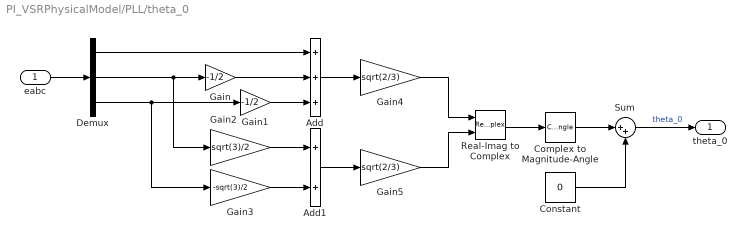
== system PI_VSRPhysicalModel/PLL/theta_0 ==
  eabc : Inport
  Add : Sum  Inputs=+++
  Add1 : Sum
  Complex to Magnitude-Angle : ComplexToMagnitudeAngle  Output=Angle
  Constant : Constant  Value=0
  Demux : Demux  Outputs=3
  Gain : Gain  Gain=-1/2
  Gain1 : Gain  Gain=-1/2
  Gain2 : Gain  Gain=sqrt(3)/2
  Gain3 : Gain  Gain=-sqrt(3)/2
  Gain4 : Gain  Gain=sqrt(2/3)
  Gain5 : Gain  Gain=sqrt(2/3)
  Real-Imag to Complex : RealImagToComplex
  Sum : Sum  Inputs=|++
  theta_0 : Outport
  wires:
  Demux/3 -> Gain1/1, Gain3/1
  Gain2/1 -> Add1/1
  Gain4/1 -> Real-Imag to Complex/1
  Constant/1 -> Sum/2
  Demux/1 -> Add/1
  Gain/1 -> Add/2
  Sum/1 -> theta_0/1  "theta_0"
  Demux/2 -> Gain/1, Gain2/1
  Gain5/1 -> Real-Imag to Complex/2
  Add1/1 -> Gain5/1
  Real-Imag to Complex/1 -> Complex to Magnitude-Angle/1
  eabc/1 -> Demux/1
  Gain1/1 -> Add/3
  Add/1 -> Gain4/1
  Gain3/1 -> Add1/2
  Complex to Magnitude-Angle/1 -> Sum/1

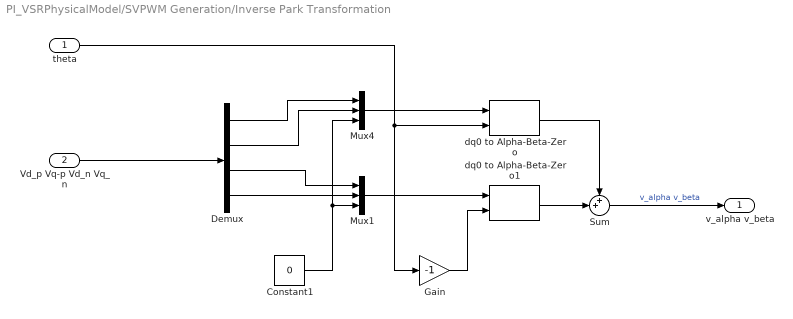
== system PI_VSRPhysicalModel/SVPWM Generation/Inverse Park Transformation ==
  theta : Inport
  Vd_p Vq-p Vd_n Vq_n : Inport  Port=2
  Constant1 : Constant  Value=0
  Demux : Demux
  Gain : Gain  Gain=-1
  Mux1 : Mux  Inputs=3
  Mux4 : Mux  Inputs=3
  Sum : Sum  Inputs=++|
  dq0 to Alpha-Beta-Zero : spsdq0toAlphaBetaZeroLib/dq0 to Alpha-Beta-Zero  Alignment=Aligned with phase A axis
      settings: SourceProductBaseCode=PS
  dq0 to Alpha-Beta-Zero1 : spsdq0toAlphaBetaZeroLib/dq0 to Alpha-Beta-Zero  Alignment=Aligned with phase A axis
      settings: SourceProductBaseCode=PS
  v_alpha v_beta : Outport
  wires:
  Demux/4 -> Mux1/2
  Demux/3 -> Mux1/1
  Mux4/1 -> dq0 to Alpha-Beta-Zero/1
  Gain/1 -> dq0 to Alpha-Beta-Zero1/2
  theta/1 -> Gain/1, dq0 to Alpha-Beta-Zero/2
  Demux/2 -> Mux4/2
  Demux/1 -> Mux4/1
  dq0 to Alpha-Beta-Zero1/1 -> Sum/2
  dq0 to Alpha-Beta-Zero/1 -> Sum/1
  Mux1/1 -> dq0 to Alpha-Beta-Zero1/1
  Constant1/1 -> Mux4/3, Mux1/3
  Vd_p Vq-p Vd_n Vq_n/1 -> Demux/1
  Sum/1 -> v_alpha v_beta/1  "v_alpha v_beta"

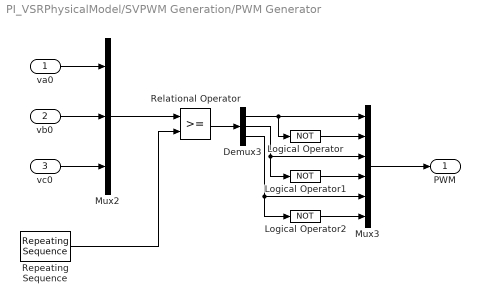
== system PI_VSRPhysicalModel/SVPWM Generation/PWM Generator ==
  va0 : Inport
  vb0 : Inport  Port=2
  vc0 : Inport  Port=3
  Demux3 : Demux  Outputs=3
  Logical Operator : Logic  Operator=NOT  AllPortsSameDT=off  OutDataTypeStr=boolean
  Logical Operator1 : Logic  Operator=NOT  AllPortsSameDT=off  OutDataTypeStr=boolean
  Logical Operator2 : Logic  Operator=NOT  AllPortsSameDT=off  OutDataTypeStr=boolean
  Mux2 : Mux  Inputs=3
  Mux3 : Mux  Inputs=6
  Relational Operator : RelationalOperator  OutDataTypeStr=boolean  RndMeth=Simplest
  Repeating Sequence : simulink/Sources/Repeating Sequence  rep_seq_t=[0 1/4 0.75 1]/f_PWM  rep_seq_y=[0 1 -1 0]
  PWM : Outport
  wires:
  Demux3/3 -> Logical Operator2/1, Mux3/5
  Demux3/1 -> Logical Operator/1, Mux3/1
  Logical Operator/1 -> Mux3/2
  Repeating Sequence/1 -> Relational Operator/2
  Demux3/2 -> Mux3/3, Logical Operator1/1
  Relational Operator/1 -> Demux3/1
  Logical Operator2/1 -> Mux3/6
  Mux2/1 -> Relational Operator/1
  Logical Operator1/1 -> Mux3/4
  Mux3/1 -> PWM/1
  vb0/1 -> Mux2/2
  vc0/1 -> Mux2/3
  va0/1 -> Mux2/1

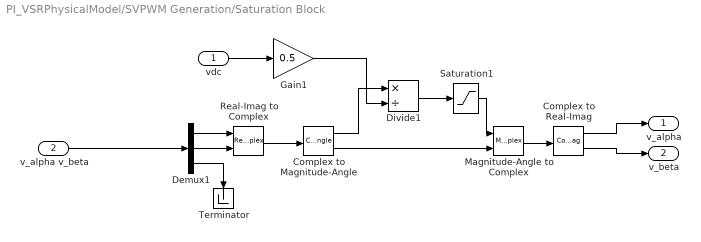
== system PI_VSRPhysicalModel/SVPWM Generation/Saturation Block ==
  vdc : Inport
  v_alpha v_beta : Inport  Port=2
  Complex to Magnitude-Angle : ComplexToMagnitudeAngle
  Complex to Real-Imag : ComplexToRealImag
  Demux1 : Demux  Outputs=3
  Divide1 : Product  Inputs=*/
  Gain1 : Gain  Gain=0.5
  Magnitude-Angle to Complex : MagnitudeAngleToComplex
  Real-Imag to Complex : RealImagToComplex
  Saturation1 : Saturate  UpperLimit=sqrt(2)  LowerLimit=-sqrt(2)
  Terminator : Terminator
  v_alpha : Outport
  v_beta : Outport  Port=2
  wires:
  Complex to Magnitude-Angle/2 -> Magnitude-Angle to Complex/2
  Real-Imag to Complex/1 -> Complex to Magnitude-Angle/1
  Saturation1/1 -> Magnitude-Angle to Complex/1
  Complex to Magnitude-Angle/1 -> Divide1/1
  vdc/1 -> Gain1/1
  Gain1/1 -> Divide1/2
  Demux1/1 -> Real-Imag to Complex/1
  Magnitude-Angle to Complex/1 -> Complex to Real-Imag/1
  Divide1/1 -> Saturation1/1
  Demux1/3 -> Terminator/1
  Demux1/2 -> Real-Imag to Complex/2
  Complex to Real-Imag/1 -> v_alpha/1
  Complex to Real-Imag/2 -> v_beta/1
  v_alpha v_beta/1 -> Demux1/1

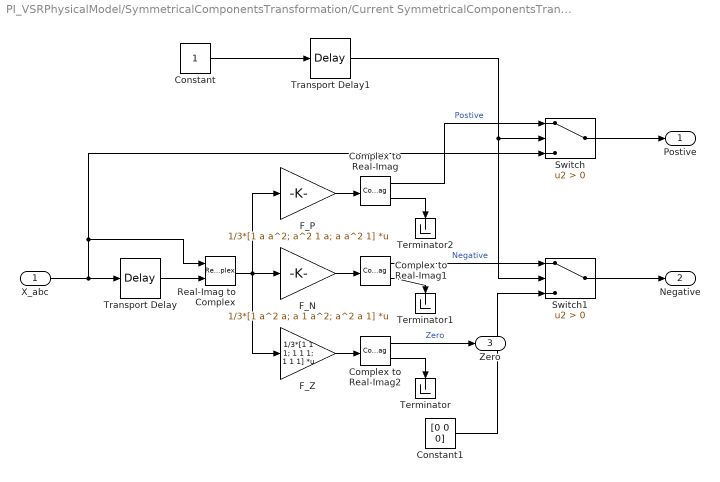
== system PI_VSRPhysicalModel/SymmetricalComponentsTransformation/Current SymmetricalComponentsTransformation ==
  X_abc : Inport
  Complex to Real-Imag : ComplexToRealImag
  Complex to Real-Imag1 : ComplexToRealImag
  Complex to Real-Imag2 : ComplexToRealImag
  Constant : Constant
  Constant1 : Constant  Value=[0 0 0]
  F_N : Gain  Gain=1/3*[1 a^2 a; a 1 a^2; a^2 a 1]  Multiplication=Matrix(K*u)
  F_P : Gain  Gain=1/3*[1 a a^2; a^2 1 a; a a^2 1]  Multiplication=Matrix(K*u)
  F_Z : Gain  Gain=1/3*[1 1 1; 1 1 1; 1 1 1]  Multiplication=Matrix(K*u)
  Real-Imag to Complex : RealImagToComplex
  Switch : Switch  Criteria=u2 > Threshold
  Switch1 : Switch  Criteria=u2 > Threshold  OutDataTypeStr=double
  Terminator : Terminator
  Terminator1 : Terminator
  Terminator2 : Terminator
  Transport Delay : TransportDelay  DelayTime=1/(4*50)  BufferSize=10000
  Transport Delay1 : TransportDelay  DelayTime=1/(4*50)  BufferSize=10000
  Postive : Outport
  Negative : Outport  Port=2
  Zero : Outport  Port=3
  wires:
  Complex to Real-Imag/1 -> Switch/1  "Postive"
  Complex to Real-Imag1/1 -> Switch1/1  "Negative"
  Complex to Real-Imag2/1 -> Zero/1  "Zero"
  X_abc/1 -> Transport Delay/1, Switch/3, Real-Imag to Complex/1
  Complex to Real-Imag/2 -> Terminator2/1
  F_Z/1 -> Complex to Real-Imag2/1
  F_N/1 -> Complex to Real-Imag1/1
  Transport Delay/1 -> Real-Imag to Complex/2
  F_P/1 -> Complex to Real-Imag/1
  Real-Imag to Complex/1 -> F_N/1, F_Z/1, F_P/1
  Complex to Real-Imag1/2 -> Terminator1/1
  Complex to Real-Imag2/2 -> Terminator/1
  Constant1/1 -> Switch1/3
  Constant/1 -> Transport Delay1/1
  Transport Delay1/1 -> Switch1/2, Switch/2
  Switch1/1 -> Negative/1
  Switch/1 -> Postive/1

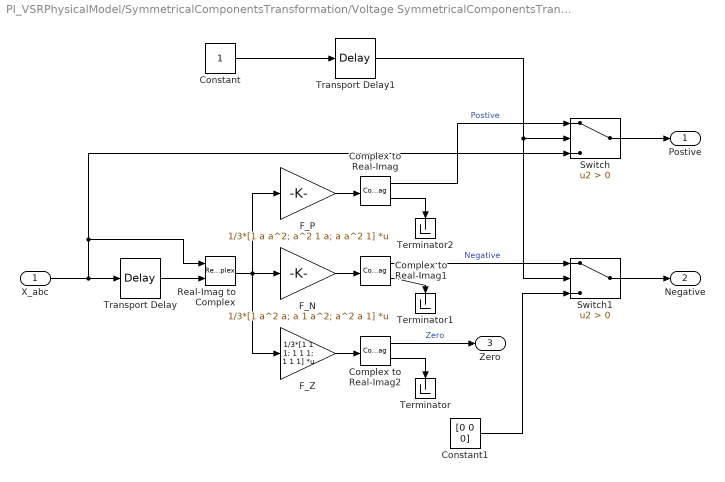
== system PI_VSRPhysicalModel/SymmetricalComponentsTransformation/Voltage SymmetricalComponentsTransformation ==
  X_abc : Inport
  Complex to Real-Imag : ComplexToRealImag
  Complex to Real-Imag1 : ComplexToRealImag
  Complex to Real-Imag2 : ComplexToRealImag
  Constant : Constant
  Constant1 : Constant  Value=[0 0 0]
  F_N : Gain  Gain=1/3*[1 a^2 a; a 1 a^2; a^2 a 1]  Multiplication=Matrix(K*u)
  F_P : Gain  Gain=1/3*[1 a a^2; a^2 1 a; a a^2 1]  Multiplication=Matrix(K*u)
  F_Z : Gain  Gain=1/3*[1 1 1; 1 1 1; 1 1 1]  Multiplication=Matrix(K*u)
  Real-Imag to Complex : RealImagToComplex
  Switch : Switch  Criteria=u2 > Threshold
  Switch1 : Switch  Criteria=u2 > Threshold
  Terminator : Terminator
  Terminator1 : Terminator
  Terminator2 : Terminator
  Transport Delay : TransportDelay  DelayTime=1/(4*50)  BufferSize=10000
  Transport Delay1 : TransportDelay  DelayTime=1/(4*50)  BufferSize=10000
  Postive : Outport
  Negative : Outport  Port=2
  Zero : Outport  Port=3
  wires:
  Complex to Real-Imag2/2 -> Terminator/1
  Complex to Real-Imag1/2 -> Terminator1/1
  Real-Imag to Complex/1 -> F_P/1, F_Z/1, F_N/1
  F_P/1 -> Complex to Real-Imag/1
  Transport Delay/1 -> Real-Imag to Complex/2
  F_N/1 -> Complex to Real-Imag1/1
  F_Z/1 -> Complex to Real-Imag2/1
  Complex to Real-Imag/2 -> Terminator2/1
  X_abc/1 -> Real-Imag to Complex/1, Switch/3, Transport Delay/1
  Complex to Real-Imag2/1 -> Zero/1  "Zero"
  Complex to Real-Imag1/1 -> Switch1/1  "Negative"
  Complex to Real-Imag/1 -> Switch/1  "Postive"
  Switch/1 -> Postive/1
  Constant/1 -> Transport Delay1/1
  Transport Delay1/1 -> Switch1/2, Switch/2
  Switch1/1 -> Negative/1
  Constant1/1 -> Switch1/3

== matlab function PI_VSRPhysicalModel/PI ctrl DC-Link Voltage Controller/MATLAB Function ==
  data: Grid_Voltages input; i_ref output; wref input
function i_ref = fcn(Grid_Voltages, wref)
    % Extract Grid Components
    Ed_p = Grid_Voltages(1); Eq_p = Grid_Voltages(2);
    Ed_n = Grid_Voltages(3); Eq_n = Grid_Voltages(4);

    D = (Ed_p^2 + Eq_p^2)-(Ed_n^2 +Eq_n^2);
    
    
    i_ref = (2*wref)/(3*D)* Grid_Voltages;

== matlab function PI_VSRPhysicalModel/PLL/V_AlphaBeta//Vdq ==
  data: valpha input; vd output; vbeta input; theta input; vq output
function [vd,vq]= fcn(valpha,vbeta,theta)

vd = (valpha*cos(theta)+vbeta*sin(theta));
vq = (-valpha*sin(theta)+vbeta*cos(theta));

== matlab function PI_VSRPhysicalModel/PLL/Vabc//V_AlphaBeta ==
  data: va input; valpha output; vb input; vc input; vbeta output
function [valpha,vbeta]= fcn(va,vb,vc)

valpha = 2/3*(va - 0.5*vb - 0.5*vc);
vbeta =  2/3*(sqrt(3)/2*vb - sqrt(3)/2*vc);

== matlab function PI_VSRPhysicalModel/PLL/ctrlGain ==
  data: ed input; gamma1 output; eq input; gamma2 output
function [gamma1,gamma2] = fcn(ed,eq)

phi = 2*pi*100;

eg = sqrt(ed^2+eq^2);

gamma1 = (phi^2)/eg;
gamma2 = (2*phi)/eg;
